simulink model "w2_warplab_buffers"  (Simulink 7.7)
settings: Solver=VariableStepDiscrete  SolverMode=SingleTasking  StartTime=0.0  StopTime=200000  RelTol=1e-3
InitFcn:
  | w2_warplab_buffers_init
StartFcn:
  | w2_warplab_buffers_init
values from neighbouring files (symbols this model uses):
  NumSamps_Rx_IQ = 2^14    (= 16384)    [w2_warplab_buffers_init.m]
  NumSamps_Rx_RSSI = 2^12    (= 4096)    [w2_warplab_buffers_init.m]
  NumSamps_Tx_IQ = 2^14    (= 16384)    [w2_warplab_buffers_init.m]
undefined symbols (not defined in the file or in its folder): gcbh, xlBlockLoadCallback, xlGetNormalizedPeriod
libraries: xbsIndex_r4 x752
(part 1 of 7)
settings Model: Creator=mduarte  LastModifiedBy=mango
settings OptimizationCC: InlineParams=on  InitFltsAndDblsToZero=on
settings DebuggingCC: SaveWithParameterizedLinksMsg=none  StrictBusMsg=Warning
settings GRTTargetCC: TargetFcnLib=ansi_tfl_tmw.mat

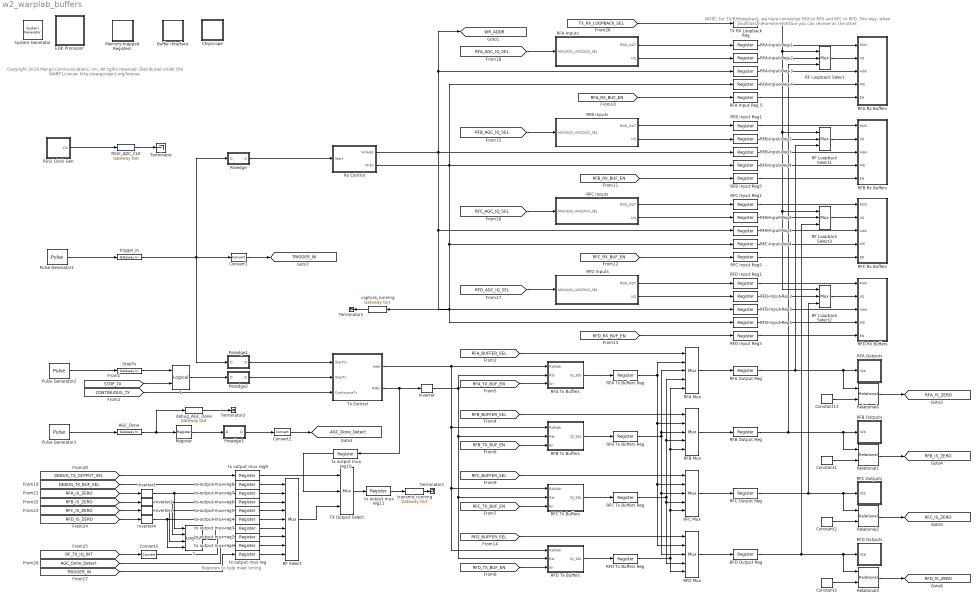
== system w2_warplab_buffers ==
  note: Copyright 2014 Mango Communications, Inc. All rights reserved.
      |
      | Distributed under the WARP License:
      | http://warpproject.org/license
  note: NOTE: For TX/RX Loopback, we have connected RFA to RFB and RFC to RFD.
      | This way, when you transmit on one interface you can receive on the other.
  note: Registers to help
      | meet timing
  " 1" : xbsIndex_r4/Logical  logical_function=OR  inputs=2  en=off  latency=0  precision=Full  arith_type=Unsigned  n_bits=16  bin_pt=0  align_bp=on  dbl_ovrd=off  block_type=logical
      settings: block_version=9.1.01
  " 2" : xbsIndex_r4/Logical  logical_function=OR  inputs=4  en=off  latency=0  precision=Full  arith_type=Unsigned  n_bits=16  bin_pt=0  align_bp=on  dbl_ovrd=off  block_type=logical
      settings: block_version=9.1.01
  " System Generator" : xbsIndex_r4/ System Generator  Tag=genX  SystemSampleTime=-1  xilinxfamily=virtex4  part=xc4vfx100  speed=-11  package=ff1517  synthesis_tool=XST  clock_wrapper=Clock Enables  directory=./warplab_buffers  proj_type=Project Navigator  Synth_file=XST Defaults  Impl_file=ISE Defaults  testbench=off  simulink_period=1  sysclk_period=10  dcm_input_clock_period=10  incr_netlist=off  trim_vbits=Everywhere in SubSystem  dbl_ovrd=According to Block Masks  core_generation=According to Block Masks  run_coregen=off  deprecated_control=off  eval_field=0  block_type=sysgen
  AGC_Done : xbsIndex_r4/Gateway In  gui_display_data_type=Fixed-point  arith_type=Unsigned  n_bits=1  bin_pt=0  preci_type=Single  exp_width=8  frac_width=24  quantization="Round  (unbiased: +/- Inf)"  overflow=Saturate  period=1  dbl_ovrd=off  timing_constraint=None  locs_specified=off  LOCs={}  UseAsADC=off  ADCChannel='1'  inherit_from_input=off  hdl_port=on  block_type=gatewayin
      settings: infoedit="Gateway in block.  Converts inputs of type Simulink integer, double and fixed point to  Xilinx fixed point type.<P><P>Hardware notes:  In hardware these blocks become top level input ports."  block_version=VER_STRING_GOES_HERE
  Buffer Interface : Subsystem
  Chipscope : Subsystem
  Constant{1..3,13} (4 alike) : xbsIndex_r4/Constant  const=0  gui_display_data_type=Fixed-point  arith_type=Unsigned  n_bits=32  bin_pt=0  preci_type=Single  exp_width=8  frac_width=24  explicit_period=off  period=1  equ=P=C  opselect=C  inp2=PCIN>>17  opr=+  inp1=P  carry=CIN  dbl_ovrd=off  block_type=constant
      settings: block_version=10.1.2
  Convert1 : xbsIndex_r4/Convert  gui_display_data_type=Boolean  arith_type=Boolean  n_bits=16  bin_pt=14  float_type=Single  exp_bits=8  fraction_bits=24  quantization=Truncate  overflow=Wrap  en=off  latency=0  dbl_ovrd=off  pipeline=off  block_type=convert
      settings: block_version=8.2
  Convert2 : xbsIndex_r4/Convert  gui_display_data_type=Fixed-point  arith_type=Boolean  n_bits=16  bin_pt=14  float_type=Single  exp_bits=8  fraction_bits=24  quantization=Truncate  overflow=Wrap  en=off  latency=0  dbl_ovrd=off  pipeline=off  block_type=convert
      settings: block_version=8.2
  Convert3 : xbsIndex_r4/Convert  gui_display_data_type=Fixed-point  arith_type=Boolean  n_bits=16  bin_pt=14  float_type=Single  exp_bits=8  fraction_bits=24  quantization=Truncate  overflow=Wrap  en=off  latency=0  dbl_ovrd=off  pipeline=off  block_type=convert
      settings: block_version=8.2
  EDK Processor : Subsystem  LoadFcn=xlBlockLoadCallback(gcbh);  mask(Xilinx EDK Processor Block){mode=EDK pcore generation, xmp=, MemVisToProc=<qt bgcolor="#FFFFFF"><div><img src="C:/Xilinx/14.4/ISE_DS/ISE/sysgen/data/images/registerplus.gif"> &lt;&lt;TX_DELAY&gt;&gt;<br></div><div><img src="C:/Xilinx/14.4/ISE_DS/ISE/sysgen/data/images/registerplus.gif"> &lt;&lt;RF_RX_IQ_BUF_RD_BYTE_OFFSET&gt;&gt;<br></div><div><img src="C:/Xilinx/14.4/ISE_DS/ISE/sysgen/data/images/registerplus.gif"> &lt;&lt;LOAD_TIMER_64_LSB&gt;&gt;<br></div><div><img src="C:/Xilinx/14.4/ISE_DS/ISE/sysgen/data/images/registerplus.gif"> &lt;&lt;RF_RX_IQ_THRESHOLD&gt;&gt;<br></div><div><img src="C:/Xilinx/14.4/ISE_DS/ISE/sysgen/data/images/registerplus.gif"> &lt;&lt;RX_LENGTH&gt;&gt;<br></div><div><img src="C:/Xilinx/14.4/ISE_DS/ISE/sysgen/data/images/registerplus.gif"> &lt;&lt;TX_LENGTH&gt;&gt;<br></div><div><img src="C:/Xilinx/14.4/ISE_DS/ISE/sysgen/data/images/registerplus.gif"> &lt;&lt;RF_RX_IQ_BUF_WR_BYTE_OFFSET&gt;&gt;<br></div><div><img src="C:/Xilinx/14.4/ISE_DS/ISE/sysgen/data/images/registerplus.gif"> &lt;&lt;RF_BUFFER_SEL&gt;&gt;<br></div><div><img src="C:/Xilinx/14.4/ISE_DS/ISE/sysgen/data/images/registerplus.gif"> &lt;&lt;RX_BUF_EN&gt;&gt;<br></div><div><img src="C:/Xilinx/14.4/ISE_DS/ISE/sysgen/data/images/registerplus.gif"> &lt;&lt;RF_TX_IQ_THRESHOLD&gt;&gt;<br></div><div><img src="C:/Xilinx/14.4/ISE_DS/ISE/sysgen/data/images/registerplus.gif"> &lt;&lt;CONFIG&gt;&gt;<br></div><div><img src="C:/Xilinx/14.4/ISE_DS/ISE/sysgen/data/images/registerplus.gif"> &lt;&lt;RF_ERROR_CLR&gt;&gt;<br></div><div><img src="C:/Xilinx/14.4/ISE_DS/ISE/sysgen/data/images/registerplus.gif"> &lt;&lt;RF_TX_IQ_BUF_WR_BYTE_OFFSET&gt;&gt;<br></div><div><img src="C:/Xilinx/14.4/ISE_DS/ISE/sysgen/data/images/registerplus.gif"> &lt;&lt;LOAD_TIMER_64_MSB&gt;&gt;<br></div><div><img src="C:/Xilinx/14.4/ISE_DS/ISE/sysgen/data/images/registerplus.gif"> &lt;&lt;TX_BUF_EN&gt;&gt;<br></div><div><img src="C:/Xilinx/14.4/ISE_DS/ISE/sysgen/data/images/registerplus.gif"> &lt;&lt;RF_TX_IQ_BUF_OCCUPANCY&gt;&gt;<br></div><div><img src="C:/Xilinx/14.4/ISE_DS/ISE/sysgen/data/images/registerplus.gif"> &lt;&lt;RF_TX_IQ_BUF_RD_BYTE_OFFSET&gt;&gt;<br></div><div><img src="C:/Xilinx/14.4/ISE_DS/ISE/sysgen/data/images/registerplus.gif"> &lt;&lt;AGC_GAINS&gt;&gt;<br></div><div><img src="C:/Xilinx/14.4/ISE_DS/ISE/sysgen/data/images/registerplus.gif"> &lt;&lt;RF_RX_IQ_BUF_OCCUPANCY&gt;&gt;<br></div><div><img src="C:/Xilinx/14.4/ISE_DS/ISE/sysgen/data/images/registerplus.gif"> &lt;&lt;RF_RX_IQ_BUF_WR_BYTE_OFFSET_UPDATE&gt;&gt;<br></div><div><img src="C:/Xilinx/14.4/ISE_DS/ISE/sysgen/data/images/registerplus.gif"> &lt;&lt;INT_STATUS&gt;&gt;<br></div><div><img src="C:/Xilinx/14.4/ISE_DS/ISE/sysgen/data/images/registerplus.gif"> &lt;&lt;BUFF_SIZES&gt;&gt;<br></div><div><img src="C:/Xilinx/14.4/ISE_DS/ISE/sysgen/data/images/registerplus.gif"> &lt;&lt;DESIGN_VER&gt;&gt;<br></div><div><img src="C:/Xilinx/14.4/ISE_DS/ISE/sysgen/data/images/registerplus.gif"> &lt;&lt;RF_TX_IQ_STATUS&gt;&gt;<br></div><div><img src="C:/Xilinx/14.4/ISE_DS/ISE/sysgen/data/images/registerplus.gif"> &lt;&lt;STATUS&gt;&gt;<br></div><div><img src="C:/Xilinx/14.4/ISE_DS/ISE/sysgen/data/images/registerplus.gif"> &lt;&lt;RFCD_AGC_DONE_RSSI&gt;&gt;<br></div><div><img src="C:/Xilinx/14.4/ISE_DS/ISE/sysgen/data/images/registerplus.gif"> &lt;&lt;RFAB_AGC_DONE_RSSI&gt;&gt;<br></div><div><img src="C:/Xilinx/14.4/ISE_DS/ISE/sysgen/data/images/registerplus.gif"> &lt;&lt;TIMER_64_MSB&gt;&gt;<br></div><div><img src="C:/Xilinx/14.4/ISE_DS/ISE/sysgen/data/images/registerplus.gif"> &lt;&lt;TIMER_64_LSB&gt;&gt;<br></div><div><img src="C:/Xilinx/14.4/ISE_DS/ISE/sysgen/data/images/registerplus.gif"> &lt;&lt;AGC_DONE_ADDR&gt;&gt;<br></div><div><img src="C:/Xilinx/14.4/ISE_DS/ISE/sysgen/data/images/memoryplus.gif"> &lt;&lt;RFD_IQ_Tx_Buffer&gt;&gt;<br></div><div><img src="C:/Xilinx/14.4/ISE_DS/ISE/sysgen/data/images/memoryplus.gif"> &lt;&lt;RFD_RSSI_Buffer&gt;&gt;<br></div><div><img src="C:/Xilinx/14.4/ISE_DS/ISE/sysgen/data/images/memoryplus.gif"> &lt;&lt;RFD_IQ_Rx_Buffer&gt;&gt;<br></div><div><img src="C:/Xilinx/14.4/ISE_DS/ISE/sysgen/data/images/memoryplus.gif"> &lt;&lt;RFC_IQ_Tx_Buffer&gt;&gt;<br></div><div><img src="C:/Xilinx/14.4/ISE_DS/ISE/sysgen/data/images/memoryplus.gif"> &lt;&lt;RFC_RSSI_Buffer&gt;&gt;<br></div><div><img src="C:/Xilinx/14.4/ISE_DS/ISE/sysgen/data/images/memoryplus.gif"> &lt;&lt;RFC_IQ_Rx_Buffer&gt;&gt;<br></div><div><img src="C:/Xilinx/14.4/ISE_DS/ISE/sysgen/data/images/memoryplus.gif"> &lt;&lt;RFB_IQ_Tx_Buffer&gt;&gt;<br></div><div><img src="C:/Xilinx/14.4/ISE_DS/ISE/sysgen/data/images/memoryplus.gif"> &lt;&lt;RFB_RSSI_Buffer&gt;&gt;<br></div><div><img src="C:/Xilinx/14.4/ISE_DS/ISE/sysgen/data/images/memoryplus.gif"> &lt;&lt;RFB_IQ_Rx_Buffer&gt;&gt;<br></div><div><img src="C:/Xilinx/14.4/ISE_DS/ISE/sysgen/data/images/memoryplus.gif"> &lt;&lt;RFA_IQ_Tx_Buffer&gt;&gt;<br></div><div><img src="C:/Xilinx/14.4/ISE_DS/ISE/sysgen/data/images/memoryplus.gif"> &lt;&lt;RFA_RSSI_Buffer&gt;&gt;<br></div><div><img src="C:/Xilinx/14.4/ISE_DS/ISE/sysgen/data/images/memoryplus.gif"> &lt;&lt;RFA_IQ_Rx_Buffer&gt;&gt;<br></div></qt>, AvailableMemories=<empty>, portInterfaceTable={'exposed'=>[],'portdir'=>[],'portname'=>[],'shortname'=>[]}, bus_type_sgadvanced=, bus_type=PLB, baseaddr=0x80000000, baseaddr_lock_sgadvanced=, baseaddr_lock=off, dual_clock_sgadvanced=, dual_clock=on, reg_readback_sgadvanced=, reg_readback=on, ucf_file=, inheritDeviceType_sgadvanced=, inheritDeviceType=off, elf_file=, codebug_sgadvanced=, codebug=on, clock_name=plb, internalPortList={}, resetPolarity=0, memxtable={'mladdr'=>[0.00000000000000000,1.00000000000000000,2.00000000000000000,3.00000000000000000,4.00000000000000000,5.00000000000000000,6.00000000000000000,7.00000000000000000,8.00000000000000000,9.00000000000000000,10.00000000000000000,11.00000000000000000,12.00000000000000000,13.00000000000000000,14.00000000000000000,0.00000000000000000,1.00000000000000000,2.00000000000000000,3.00000000000000000,4.00000000000000000,5.00000000000000000,6.00000000000000000,7.00000000000000000,8.00000000000000000,9.00000000000000000,10.00000000000000000,11.00000000000000000,12.00000000000000000,13.00000000000000000,14.00000000000000000,-1.00000000000000000,-1.00000000000000000,-1.00000000000000000,-1.00000000000000000,-1.00000000000000000,-1.00000000000000000,-1.00000000000000000,-1.00000000000000000,-1.00000000000000000,-1.00000000000000000,-1.00000000000000000,-1.00000000000000000],'mlist'=>['w2_warplab_buffers/Memory-mapped Registers/TxDelay','w2_warplab_buffers/Memory-mapped Registers/From Register9','w2_warplab_buffers/Memory-mapped Registers/From Register8','w2_warplab_buffers/Memory-mapped Registers/From Register7','w2_warplab_buffers/Memory-mapped Registers/From Register6','w2_warplab_buffers/Memory-mapped Registers/From Register5','w2_warplab_buffers/Memory-mapped Registers/From Register4','w2_warplab_buffers/Memory-mapped Registers/From Register2','w2_warplab_buffers/Memory-mapped Registers/From Register16','w2_warplab_buffers/Memory-mapped Registers/From Register14','w2_warplab_buffers/Memory-mapped Registers/From Register13','w2_warplab_buffers/Memory-mapped Registers/From Register12','w2_warplab_buffers/Memory-mapped Registers/From Register11','w2_warplab_buffers/Memory-mapped Registers/From Register10','w2_warplab_buffers/Memory-mapped Registers/From Register1','w2_warplab_buffers/Memory-mapped Registers/To Register9','w2_warplab_buffers/Memory-mapped Registers/To Register8','w2_warplab_buffers/Memory-mapped Registers/To Register7','w2_warplab_buffers/Memory-mapped Registers/To Register6','w2_warplab_buffers/Memory-mapped Registers/To Register5','w2_warplab_buffers/Memory-mapped Registers/To Register4','w2_warplab_buffers/Memory-mapped Registers/To Register3','w2_warplab_buffers/Memory-mapped Registers/To Register2','w2_warplab_buffers/Memory-mapped Registers/To Register10','w2_warplab_buffers/Memory-mapped Registers/To Register1','w2_warplab_buffers/Memory-mapped Registers/Radio3AGCDoneRSSI','w2_warplab_buffers/Memory-mapped Registers/Radio1AGCDoneRSSI','w2_warplab_buffers/Memory-mapped Registers/AGCDoneAddr2','w2_warplab_buffers/Memory-mapped Registers/AGCDoneAddr1','w2_warplab_buffers/Memory-mapped Registers/AGCDoneAddr','w2_warplab_buffers/Buffer Interface/RFD Buffers/Shared Memory2','w2_warplab_buffers/Buffer Interface/RFD Buffers/Shared Memory1','w2_warplab_buffers/Buffer Interface/RFD Buffers/Shared Memory','w2_warplab_buffers/Buffer Interface/RFC Buffers/Shared Memory2','w2_warplab_buffers/Buffer Interface/RFC Buffers/Shared Memory1','w2_warplab_buffers/Buffer Interface/RFC Buffers/Shared Memory','w2_warplab_buffers/Buffer Interface/RFB Buffers/Shared Memory2','w2_warplab_buffers/Buffer Interface/RFB Buffers/Shared Memory1','w2_warplab_buffers/Buffer Interface/RFB Buffers/Shared Memory','w2_warplab_buffers/Buffer Interface/RFA Buffers/Shared Memory2','w2_warplab_buffers/Buffer Interface/RFA Buffers/Shared Memory1','w2_warplab_buffers/Buffer Interface/RFA Buffers/Shared Memory'],'mlname'=>['\\'TX_DELAY\\'','\\'RF_RX_IQ_BUF_RD_BYTE_OFFSET\\'','\\'LOAD_TIMER_64_LSB\\'','\\'RF_RX_IQ_THRESHOLD\\'','\\'RX_LENGTH\\'','\\'TX_LENGTH\\'','\\'RF_RX_IQ_BUF_WR_BYTE_OFFSET\\'','\\'RF_BUFFER_SEL\\'','\\'RX_BUF_EN\\'','\\'RF_TX_IQ_THRESHOLD\\'','\\'CONFIG\\'','\\'RF_ERROR_CLR\\'','\\'RF_TX_IQ_BUF_WR_BYTE_OFFSET\\'','\\'LOAD_TIMER_64_MSB\\'','\\'TX_BUF_EN\\'','\\'RF_TX_IQ_BUF_OCCUPANCY\\'','\\'RF_TX_IQ_BUF_RD_BYTE_OFFSET\\'','\\'AGC_GAINS\\'','\\'RF_RX_IQ_BUF_OCCUPANCY\\'','\\'RF_RX_IQ_BUF_WR_BYTE_OFFSET_UPDATE\\'','\\'INT_STATUS\\'','\\'BUFF_SIZES\\'','\\'DESIGN_VER\\'','\\'RF_TX_IQ_STATUS\\'','\\'STATUS\\'','\\'RFCD_AGC_DONE_RSSI\\'','\\'RFAB_AGC_DONE_RSSI\\'','\\'TIMER_64_MSB\\'','\\'TIMER_64_LSB\\'','\\'AGC_DONE_ADDR\\'','\\'RFD_IQ_Tx_Buffer\\'','\\'RFD_RSSI_Buffer\\'','\\'RFD_IQ_Rx_Buffer\\'','\\'RFC_IQ_Tx_Buffer\\'','\\'RFC_RSSI_Buffer\\'','\\'RFC_IQ_Rx_Buffer\\'','\\'RFB_IQ_Tx_Buffer\\'','\\'RFB_RSSI_Buffer\\'','\\'RFB_IQ_Rx_Buffer\\'','\\'RFA_IQ_Tx_Buffer\\'','\\'RFA_RSSI_Buffer\\'','\\'RFA_IQ_Rx_Buffer\\''],'mlstate'=>[0.00000000000000000,0.00000000000000000,0.00000000000000000,0.00000000000000000,0.00000000000000000,0.00000000000000000,0.00000000000000000,0.00000000000000000,0.00000000000000000,0.00000000000000000,0.00000000000000000,0.00000000000000000,0.00000000000000000,0.00000000000000000,0.00000000000000000,0.00000000000000000,0.00000000000000000,0.00000000000000000,0.00000000000000000,0.00000000000000000,0.00000000000000000,0.00000000000000000,0.00000000000000000,0.00000000000000000,0.00000000000000000,0.00000000000000000,0.00000000000000000,0.00000000000000000,0.00000000000000000,0.00000000000000000,0.00000000000000000,0.00000000000000000,0.00000000000000000,0.00000000000000000,0.00000000000000000,0.00000000000000000,0.00000000000000000,0.00000000000000000,0.00000000000000000,0.00000000000000000,0.00000000000000000,0.00000000000000000]}, procinfo={}, memmapdirty=off, blockname=, xpsintstyle=default, has_advanced_control=0, sggui_pos=-1,-1,-1,-1, block_type=edkprocessor, block_version=2.7, sg_icon_stat=62,64,-1,-1,white,blue,0,07734,right,,[ ],[ ], sg_mask_display=|, sg_list_contents={'table'=>{'AvailableMemories'=>'popup(<empty>)'}}, sg_blockgui_xml=}
      mask sg_mask_display=|
      | fprintf('','COMMENT: begin icon graphics');
      | patch([0 62 62 0 0 ],[0 0 64 64 0 ],[0.77 0.82 0.91 ]);
      | plot([0 62 62 0 0 ],[0 0 64 64 0 ]);
      | patch([13.2 24.76 32.76 40.76 48.76 32.76 21.2 13.2 ],[40.88 40.88 48.88 40.88 48.88 48.88 48.88 40.88 ],[1 1 1 ]);
      | patch([21.2 32.76 24.76 13.2 21.2 ],[32.88 32.88 40.88 40.88 32.88 ],[0.931 0.946 0.973 ]);
      | patch([13.2 24.76 32.76 21.2 13.2 ],[24.88 24.88 32.88 32.88 24.88 ],[1 1 1 ]);
      | patch([21.2 48.76 40.76 32.76 24.76 13.2 21.2 ],[16.88 16.88 24.88 16.88 24.88 24.88 16.88 ],[0.931 0.946 0.973 ]);
      | fprintf('','COMMENT: end icon graphics');
      | fprintf('','COMMENT: begin icon text');
      | fprintf('','COMMENT: end icon text');
      mask prompts: mode "Configure Processor for"; xmp "XPS Project"; MemVisToProc ""; AvailableMemories "Available Memories"; portInterfaceTable ""; bus_type_sgadvanced ""; bus_type "Bus Type"; baseaddr "Base Address"; baseaddr_lock_sgadvanced ""; baseaddr_lock "Lock"; dual_clock_sgadvanced ""; dual_clock "Dual Clocks"; reg_readback_sgadvanced ""; reg_readback "Register Read-Back"; ucf_file "Constraint File"; inheritDeviceType_sgadvanced ""; inheritDeviceType "Inherit Device Type"; elf_file "Initial Program"; codebug_sgadvanced ""; codebug "Enable Co-Debug with Xilinx SDK (Beta)"; clock_name ""; internalPortList ""; resetPolarity ""; memxtable ""; procinfo ""; memmapdirty ""; blockname ""; xpsintstyle ""; has_advanced_control ""; sggui_pos ""; block_type ""; block_version ""; sg_icon_stat ""; sg_mask_display ""; sg_list_contents ""; sg_blockgui_xml ""
      mask help: Xilinx EDK Processor
      mask init:
      | try
      |   tmp_gcb = gcb;
      |   tmp_gcbh = gcbh;
      |   if (strcmp('SysGenIndex',get_param(bdroot(tmp_gcbh),'tag')) && ~isempty(regexp(bdroot(tmp_gcb), '^xbs', 'once')))
      |     return;
      |   end;
      |   xlMungeMaskParams;
      | 
      |   block_type='edkprocessor';
      | 
      |   serialized_declarations = '{''block_type''=>''String''}';
      |   xledkprocessor_init();
      |   ptable_ = xlblockprep(get_param(tmp_gcb, 'MaskWSVariables'));
      |   try
      |     xlBlockMoveCallback(tmp_gcbh);
      |   catch 
      |      clear global xl_updateicon_recursion_guard;
      |   end;
      | catch
      |   global dbgsysgen;
      |   if(~isempty(dbgsysgen) && dbgsysgen)
      |     e = regexprep(lasterr, '\n', '\nError: ');
      |     disp(['Error: While running MaskInit code on block ' tmp_gcb ': ' e]);
      |     error(e);
      |   end
      | end
      settings: CopyFcn=xlProcBlockCopyCallback(gcbh);xlBlockMoveCallback(gcbh);  DeleteFcn=xlDestroyGui(gcbh);  ModelCloseFcn=xlDestroyGui(gcbh);  PreSaveFcn=xlBlockPreSaveCallback(gcbh);  PostSaveFcn=xlBlockPostSaveCallback(gcbh);  DestroyFcn=xlDestroyGui(gcbh);  OpenFcn=bh=gcbh;xlProcBlockCallbacks('populatesharedmemorylistbox',bh);xlOpenGui(bh, 'edkprocessor_gui.xml', @xlProcBlockEnablement, @xlProcBlockAction);  CloseFcn=xlDestroyGui(gcbh);  MoveFcn=xlBlockMoveCallback(gcbh);
      mask Help: eval('');xlDoc('-book','sysgen','-topic','EDK_Processor');
      mask StyleString: popup(EDK pcore generation|HDL netlisting),edit,edit,edit,edit,edit,popup(AXI|PLB),edit,edit,checkbox,edit,checkbox,edit,checkbox,edit,edit,checkbox,edit,edit,checkbox,edit,edit,edit,edit,edit,edit,edit,edit,edit,edit,edit,edit,edit,edit,edit,edit
      mask Display:
      | fprintf('','COMMENT: begin icon graphics');
      | patch([0 62 62 0 0 ],[0 0 64 64 0 ],[0.77 0.82 0.91 ]);
      | plot([0 62 62 0 0 ],[0 0 64 64 0 ]);
      | patch([13.2 24.76 32.76 40.76 48.76 32.76 21.2 13.2 ],[40.88 40.88 48.88 40.88 48.88 48.88 48.88 40.88 ],[1 1 1 ]);
      | patch([21.2 32.76 24.76 13.2 21.2 ],[32.88 32.88 40.88 40.88 32.88 ],[0.931 0.946 0.973 ]);
      | patch([13.2 24.76 32.76 21.2 13.2 ],[24.88 24.88 32.88 32.88 24.88 ],[1 1 1 ]);
      | patch([21.2 48.76 40.76 32.76 24.76 13.2 21.2 ],[16.88 16.88 24.88 16.88 24.88 24.88 16.88 ],[0.931 0.946 0.973 ]);
      | fprintf('','COMMENT: end icon graphics');
      | fprintf('','COMMENT: begin icon text');
      | disp('');
      | 
      | fprintf('','COMMENT: end icon text');
  Inverter{,1..4} (5 alike) : xbsIndex_r4/Inverter  en=off  latency=0  dbl_ovrd=off  block_type=inv
      settings: block_version=8.2
  Memory-mapped Registers : Subsystem
  Posedge : Subsystem
  Posedge1 : Subsystem
  Posedge2 : Subsystem
  Posedge3 : Subsystem
  Pulse Generator1 : DiscretePulseGenerator  Period=2^20  PulseWidth=50  PhaseDelay=100
  Pulse Generator2 : DiscretePulseGenerator  Period=10 * 2^14  PulseWidth=50  PhaseDelay=2.5 * 2^14
  Pulse Generator3 : DiscretePulseGenerator  Period=20000  PulseWidth=50  PhaseDelay=374
  RF Loopback Select{,1..3} (4 alike) : xbsIndex_r4/Mux  inputs=2  en=off  latency=0  precision=Full  arith_type=Unsigned  n_bits=16  bin_pt=14  quantization=Truncate  overflow=Wrap  dbl_ovrd=off  block_type=mux
  RF Select : xbsIndex_r4/Mux  inputs=8  en=off  latency=0  precision=Full  arith_type=Unsigned  n_bits=16  bin_pt=14  quantization=Truncate  overflow=Wrap  dbl_ovrd=off  block_type=mux
  RFA Rx Buffers : Subsystem
  RFA Input Reg {1..5} (5 alike) : xbsIndex_r4/Register  init=0  rst=off  en=off  dbl_ovrd=off  block_type=register
  RFA Inputs : Subsystem
  RFA Mux : xbsIndex_r4/Mux  inputs=4  en=off  latency=0  precision=Full  arith_type=Unsigned  n_bits=16  bin_pt=14  quantization=Truncate  overflow=Wrap  dbl_ovrd=off  block_type=mux
  "RFA Output Reg " : xbsIndex_r4/Register  init=0  rst=off  en=off  dbl_ovrd=off  block_type=register
  RFA Outputs : Subsystem
  RFA Tx Buffers : Subsystem
  RFA Tx Buffers Reg : xbsIndex_r4/Register  init=0  rst=off  en=off  dbl_ovrd=off  block_type=register
  RFB Rx Buffers : Subsystem
  RFB Input Reg{1..5} (5 alike) : xbsIndex_r4/Register  init=0  rst=off  en=off  dbl_ovrd=off  block_type=register
  RFB Inputs : Subsystem
  RFB Mux : xbsIndex_r4/Mux  inputs=4  en=off  latency=0  precision=Full  arith_type=Unsigned  n_bits=16  bin_pt=14  quantization=Truncate  overflow=Wrap  dbl_ovrd=off  block_type=mux
  RFB Output Reg : xbsIndex_r4/Register  init=0  rst=off  en=off  dbl_ovrd=off  block_type=register
  RFB Outputs : Subsystem
  RFB Tx Buffers : Subsystem
  RFB Tx Buffers Reg : xbsIndex_r4/Register  init=0  rst=off  en=off  dbl_ovrd=off  block_type=register
  RFC Rx Buffers : Subsystem
  RFC Input Reg{1..5} (5 alike) : xbsIndex_r4/Register  init=0  rst=off  en=off  dbl_ovrd=off  block_type=register
  RFC Inputs : Subsystem
  RFC Mux : xbsIndex_r4/Mux  inputs=4  en=off  latency=0  precision=Full  arith_type=Unsigned  n_bits=16  bin_pt=14  quantization=Truncate  overflow=Wrap  dbl_ovrd=off  block_type=mux
  RFC Output Reg : xbsIndex_r4/Register  init=0  rst=off  en=off  dbl_ovrd=off  block_type=register
  RFC Outputs : Subsystem
  RFC Tx Buffers : Subsystem
  RFC Tx Buffers Reg : xbsIndex_r4/Register  init=0  rst=off  en=off  dbl_ovrd=off  block_type=register
  RFD Rx Buffers : Subsystem
  RFD Input Reg{1..5} (5 alike) : xbsIndex_r4/Register  init=0  rst=off  en=off  dbl_ovrd=off  block_type=register
  RFD Inputs : Subsystem
  RFD Mux : xbsIndex_r4/Mux  inputs=4  en=off  latency=0  precision=Full  arith_type=Unsigned  n_bits=16  bin_pt=14  quantization=Truncate  overflow=Wrap  dbl_ovrd=off  block_type=mux
  RFD Output Reg : xbsIndex_r4/Register  init=0  rst=off  en=off  dbl_ovrd=off  block_type=register
  RFD Outputs : Subsystem
  RFD Tx Buffers : Subsystem
  RFD Tx Buffers Reg : xbsIndex_r4/Register  init=0  rst=off  en=off  dbl_ovrd=off  block_type=register
  RSSI Clock Gen : Subsystem
  RSSI_ADC_CLK : xbsIndex_r4/Gateway Out  inherit_from_input=off  hdl_port=on  timing_constraint=None  locs_specified=off  LOCs={}  UseAsDAC=off  DACChannel='1'  block_type=gatewayout
      settings: infoedit="Gateway out block.  Converts Xilinx fixed point inputs into ouputs of type Simulink integer, double, or fixed point.<P><P>Hardware notes:  In hardware these blocks become top level output ports or are discarded, depending on how they are configured."  block_version=8.2
  Register : xbsIndex_r4/Register  init=0  rst=off  en=off  dbl_ovrd=off  block_type=register
      settings: block_version=8.2
  Relational{1..3,6} (4 alike) : xbsIndex_r4/Relational  mode=a=b  en=off  latency=0  dbl_ovrd=off  block_type=relational
      settings: block_version=8.2
  Rx Control : Subsystem
  StopTx : xbsIndex_r4/Gateway In  gui_display_data_type=Fixed-point  arith_type=Unsigned  n_bits=1  bin_pt=0  preci_type=Single  exp_width=8  frac_width=24  quantization="Round  (unbiased: +/- Inf)"  overflow=Saturate  period=1  dbl_ovrd=off  timing_constraint=None  locs_specified=off  LOCs={}  UseAsADC=off  ADCChannel='1'  inherit_from_input=off  hdl_port=on  block_type=gatewayin
      settings: block_version=VER_STRING_GOES_HERE
  TX Output Select : xbsIndex_r4/Mux  inputs=2  en=off  latency=0  precision=Full  arith_type=Unsigned  n_bits=16  bin_pt=14  quantization=Truncate  overflow=Wrap  dbl_ovrd=off  block_type=mux
  TX RX Loopback Reg : xbsIndex_r4/Register  init=0  rst=off  en=off  dbl_ovrd=off  block_type=register
  Terminator{,1..3} (4 alike) : Terminator
  Tx Control : Subsystem
  capture_running : xbsIndex_r4/Gateway Out  inherit_from_input=off  hdl_port=on  timing_constraint=None  locs_specified=off  LOCs={}  UseAsDAC=off  DACChannel='1'  block_type=gatewayout
      settings: infoedit="Gateway out block.  Converts Xilinx fixed point inputs into ouputs of type Simulink integer, double, or fixed point.<P><P>Hardware notes:  In hardware these blocks become top level output ports or are discarded, depending on how they are configured."  block_version=8.2
  debug_AGC_Done : xbsIndex_r4/Gateway Out  inherit_from_input=off  hdl_port=on  timing_constraint=None  locs_specified=off  LOCs={}  UseAsDAC=off  DACChannel='1'  block_type=gatewayout
      settings: block_version=8.2
  transmit_running : xbsIndex_r4/Gateway Out  inherit_from_input=off  hdl_port=on  timing_constraint=None  locs_specified=off  LOCs={}  UseAsDAC=off  DACChannel='1'  block_type=gatewayout
      settings: infoedit="Gateway out block.  Converts Xilinx fixed point inputs into ouputs of type Simulink integer, double, or fixed point.<P><P>Hardware notes:  In hardware these blocks become top level output ports or are discarded, depending on how they are configured."  block_version=8.2
  trigger_in : xbsIndex_r4/Gateway In  gui_display_data_type=Fixed-point  arith_type=Unsigned  n_bits=1  bin_pt=0  preci_type=Single  exp_width=8  frac_width=24  quantization="Round  (unbiased: +/- Inf)"  overflow=Saturate  period=1  dbl_ovrd=off  timing_constraint=None  locs_specified=off  LOCs={}  UseAsADC=off  ADCChannel='1'  inherit_from_input=off  hdl_port=on  block_type=gatewayin
      settings: infoedit="Gateway in block.  Converts inputs of type Simulink integer, double and fixed point to  Xilinx fixed point type.<P><P>Hardware notes:  In hardware these blocks become top level input ports."  block_version=VER_STRING_GOES_HERE
  tx output mux reg{,1..11} (12 alike) : xbsIndex_r4/Register  init=0  rst=off  en=off  dbl_ovrd=off  block_type=register
  tag scope: AGC_Done_Detect=global, RFA_IS_ZERO=global, RFB_IS_ZERO=global, RFC_IS_ZERO=global, RFD_IS_ZERO=global, TRIGGER_IN=global, WR_ADDR=global
  wires:
  [RFC_RX_BUF_EN] -> RFC Input Reg5/1
  [RFB_RX_BUF_EN] -> RFB Input Reg5/1
  Posedge/1(Q) -> Rx Control/1(Start)
  [RFA_RX_BUF_EN] -> RFA Input Reg 5/1
  [RFD_RX_BUF_EN] -> RFD Input Reg5/1
  Rx Control/1(WrAddr) -> RFC Input Reg3/1, RFD Input Reg3/1, [WR_ADDR], RFA Input Reg 3/1, RFB Input Reg3/1
  Rx Control/2(WrEn) -> capture_running/1, RFD Input Reg4/1, RFC Input Reg4/1, RFB Input Reg4/1, RFA Input Reg 4/1
  Posedge1/1(Q) -> Tx Control/1(StartTx)
  [CONTINUOUS_TX] -> Tx Control/3(ContinuousTx)
  Posedge2/1(Q) -> Tx Control/2(StopTx)
  " 1"/1 -> Posedge2/1(D)
  StopTx/1 -> " 1"/1
  Pulse Generator2/1 -> StopTx/1
  [RFB_TX_BUF_EN] -> RFB Tx Buffers/3(En)
  Tx Control/2(RdEn) -> Inverter/1, tx output mux reg10/1
  [RFC_TX_BUF_EN] -> RFC Tx Buffers/3(En)
  [RFA_TX_BUF_EN] -> RFA Tx Buffers/3(En)
  [RFD_TX_BUF_EN] -> RFD Tx Buffers/3(En)
  Tx Control/1(Addr) -> RFC Tx Buffers/1(RdAddr), RFD Tx Buffers/1(RdAddr), RFB Tx Buffers/1(RdAddr), RFA Tx Buffers/1(RdAddr)
  Inverter/1 -> RFC Tx Buffers/2(Rst), RFD Tx Buffers/2(Rst), RFB Tx Buffers/2(Rst), RFA Tx Buffers/2(Rst)
  [STOP_TX] -> " 1"/2
  AGC_Done/1 -> debug_AGC_Done/1, Register/1
  Pulse Generator3/1 -> AGC_Done/1
  Register/1 -> Posedge3/1(D)
  Posedge3/1(Q) -> Convert2/1
  Convert2/1 -> [AGC_Done_Detect]
  capture_running/1 -> Terminator2/1
  transmit_running/1 -> Terminator1/1
  RFA Inputs/1(RSSI_OUT) -> RFA Input Reg 1/1
  RFB Inputs/1(RSSI_OUT) -> RFB Input Reg1/1
  RFC Inputs/1(RSSI_OUT) -> RFC Input Reg1/1
  RFD Inputs/1(RSSI_OUT) -> RFD Input Reg1/1
  trigger_in/1 -> Posedge1/1(D), Posedge/1(D), Convert1/1
  RSSI_ADC_CLK/1 -> Terminator/1
  RSSI Clock Gen/1(Clk) -> RSSI_ADC_CLK/1
  Pulse Generator1/1 -> trigger_in/1
  RFA Tx Buffers/1(IQ_32b) -> RFA Tx Buffers Reg/1
  RFB Tx Buffers/1(IQ_32b) -> RFB Tx Buffers Reg/1
  RFC Tx Buffers/1(IQ_32b) -> RFC Tx Buffers Reg/1
  RFD Tx Buffers/1(IQ_32b) -> RFD Tx Buffers Reg/1
  "RFA Output Reg "/1 -> RFA Outputs/1(32b), Relational6/1, RF Loopback Select1/3
  RFB Output Reg/1 -> RFB Outputs/1(32b), Relational1/1, RF Loopback Select/3
  RFC Output Reg/1 -> RFC Outputs/1(32b), Relational2/1, RF Loopback Select2/3
  RFD Output Reg/1 -> RFD Outputs/1(32b), Relational3/1, RF Loopback Select3/3
  RFD Mux/1 -> RFD Output Reg/1
  RFC Mux/1 -> RFC Output Reg/1
  RFB Mux/1 -> RFB Output Reg/1
  RFA Mux/1 -> "RFA Output Reg "/1
  [RFA_BUFFER_SEL] -> RFA Mux/1
  [RFB_BUFFER_SEL] -> RFB Mux/1
  [RFC_BUFFER_SEL] -> RFC Mux/1
  [RFD_BUFFER_SEL] -> RFD Mux/1
  debug_AGC_Done/1 -> Terminator3/1
  [RFA_AGC_IQ_SEL] -> RFA Inputs/1(MGCAGC_AGCDCO_SEL)
  [RFB_AGC_IQ_SEL] -> RFB Inputs/1(MGCAGC_AGCDCO_SEL)
  [RFC_AGC_IQ_SEL] -> RFC Inputs/1(MGCAGC_AGCDCO_SEL)
  [RFD_AGC_IQ_SEL] -> RFD Inputs/1(MGCAGC_AGCDCO_SEL)
  Constant13/1 -> Relational6/2
  Relational6/1 -> [RFA_IS_ZERO]
  [DEBUG_TX_OUTPUT_SEL] -> tx output mux reg9/1
  RF Select/1 -> TX Output Select/3
  Constant1/1 -> Relational1/2
  Relational1/1 -> [RFB_IS_ZERO]
  Constant2/1 -> Relational2/2
  Relational2/1 -> [RFC_IS_ZERO]
  Constant3/1 -> Relational3/2
  Relational3/1 -> [RFD_IS_ZERO]
  [DEBUG_TX_BUF_SEL] -> tx output mux reg8/1
  [RFA_IS_ZERO] -> Inverter1/1
  [RFB_IS_ZERO] -> Inverter2/1
  [RFC_IS_ZERO] -> Inverter3/1
  [RFD_IS_ZERO] -> Inverter4/1
  Inverter1/1 -> " 2"/1, tx output mux reg7/1
  Inverter2/1 -> " 2"/2, tx output mux reg6/1
  Inverter3/1 -> " 2"/3, tx output mux reg5/1
  Inverter4/1 -> " 2"/4, tx output mux reg4/1
  RFA Tx Buffers Reg/1 -> RFA Mux/2, RFB Mux/2, RFC Mux/2, RFD Mux/2
  RFB Tx Buffers Reg/1 -> RFA Mux/3, RFC Mux/3, RFD Mux/3, RFB Mux/3
  RFC Tx Buffers Reg/1 -> RFA Mux/4, RFB Mux/4, RFC Mux/4, RFD Mux/4
  RFD Tx Buffers Reg/1 -> RFD Mux/5, RFC Mux/5, RFA Mux/5, RFB Mux/5
  " 2"/1 -> tx output mux reg3/1
  [RF_TX_IQ_INT] -> Convert3/1
  [AGC_Done_Detect] -> tx output mux reg1/1
  [TRIGGER_IN] -> tx output mux reg/1
  Convert1/1 -> [TRIGGER_IN]
  [TX_RX_LOOPBACK_SEL] -> TX RX Loopback Reg/1
  RFA Inputs/2(I/Q) -> RFA Input Reg 2/1
  RF Loopback Select/1 -> RFA Rx Buffers/2(I/Q)
  RF Loopback Select1/1 -> RFB Rx Buffers/2(I/Q)
  RFB Inputs/2(I/Q) -> RFB Input Reg2/1
  RFC Inputs/2(I/Q) -> RFC Input Reg2/1
  RFD Inputs/2(I/Q) -> RFD Input Reg2/1
  RFB Input Reg2/1 -> RF Loopback Select1/2
  RFA Input Reg 2/1 -> RF Loopback Select/2
  TX RX Loopback Reg/1 -> RF Loopback Select/1, RF Loopback Select1/1, RF Loopback Select3/1, RF Loopback Select2/1
  RFA Input Reg 1/1 -> RFA Rx Buffers/1(RSSI)
  RFA Input Reg 3/1 -> RFA Rx Buffers/3(Addr)
  RFA Input Reg 4/1 -> RFA Rx Buffers/4(WE)
  RFA Input Reg 5/1 -> RFA Rx Buffers/5(EN)
  RFB Input Reg1/1 -> RFB Rx Buffers/1(RSSI)
  RFB Input Reg3/1 -> RFB Rx Buffers/3(Addr)
  RFB Input Reg4/1 -> RFB Rx Buffers/4(WE)
  RFB Input Reg5/1 -> RFB Rx Buffers/5(EN)
  tx output mux reg/1 -> RF Select/9
  tx output mux reg1/1 -> RF Select/8
  tx output mux reg2/1 -> RF Select/7
  tx output mux reg3/1 -> RF Select/6
  tx output mux reg4/1 -> RF Select/5
  tx output mux reg5/1 -> RF Select/4
  tx output mux reg6/1 -> RF Select/3
  tx output mux reg7/1 -> RF Select/2
  tx output mux reg8/1 -> RF Select/1
  tx output mux reg9/1 -> TX Output Select/1
  tx output mux reg10/1 -> TX Output Select/2
  TX Output Select/1 -> tx output mux reg11/1
  tx output mux reg11/1 -> transmit_running/1
  Convert3/1 -> tx output mux reg2/1
  RFC Input Reg1/1 -> RFC Rx Buffers/1(RSSI)
  RFC Input Reg3/1 -> RFC Rx Buffers/3(Addr)
  RFC Input Reg4/1 -> RFC Rx Buffers/4(WE)
  RFC Input Reg5/1 -> RFC Rx Buffers/5(EN)
  RFD Input Reg1/1 -> RFD Rx Buffers/1(RSSI)
  RFD Input Reg3/1 -> RFD Rx Buffers/3(Addr)
  RFD Input Reg4/1 -> RFD Rx Buffers/4(WE)
  RFD Input Reg5/1 -> RFD Rx Buffers/5(EN)
  RF Loopback Select3/1 -> RFC Rx Buffers/2(I/Q)
  RF Loopback Select2/1 -> RFD Rx Buffers/2(I/Q)
  RFC Input Reg2/1 -> RF Loopback Select3/2
  RFD Input Reg2/1 -> RF Loopback Select2/2

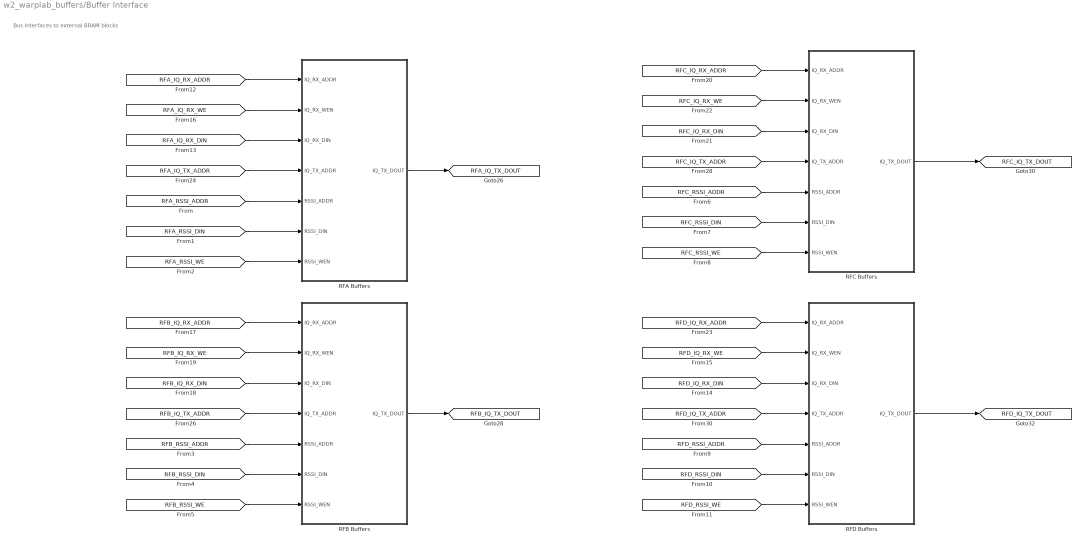
== system w2_warplab_buffers/Buffer Interface ==
  note: Bus Interfaces to external BRAM blocks
  RFA Buffers : Subsystem
  RFB Buffers : Subsystem
  RFC Buffers : Subsystem
  RFD Buffers : Subsystem
  tag scope: RFA_IQ_TX_DOUT=global, RFB_IQ_TX_DOUT=global, RFC_IQ_TX_DOUT=global, RFD_IQ_TX_DOUT=global
  wires:
  [RFA_RSSI_ADDR] -> RFA Buffers/5(RSSI_ADDR)
  [RFA_RSSI_DIN] -> RFA Buffers/6(RSSI_DIN)
  [RFA_RSSI_WE] -> RFA Buffers/7(RSSI_WEN)
  RFA Buffers/1(IQ_TX_DOUT) -> [RFA_IQ_TX_DOUT]
  [RFA_IQ_RX_ADDR] -> RFA Buffers/1(IQ_RX_ADDR)
  [RFA_IQ_RX_WE] -> RFA Buffers/2(IQ_RX_WEN)
  [RFA_IQ_RX_DIN] -> RFA Buffers/3(IQ_RX_DIN)
  [RFA_IQ_TX_ADDR] -> RFA Buffers/4(IQ_TX_ADDR)
  [RFB_IQ_RX_ADDR] -> RFB Buffers/1(IQ_RX_ADDR)
  [RFB_IQ_RX_WE] -> RFB Buffers/2(IQ_RX_WEN)
  [RFB_IQ_RX_DIN] -> RFB Buffers/3(IQ_RX_DIN)
  [RFB_IQ_TX_ADDR] -> RFB Buffers/4(IQ_TX_ADDR)
  [RFB_RSSI_ADDR] -> RFB Buffers/5(RSSI_ADDR)
  [RFB_RSSI_DIN] -> RFB Buffers/6(RSSI_DIN)
  [RFB_RSSI_WE] -> RFB Buffers/7(RSSI_WEN)
  RFB Buffers/1(IQ_TX_DOUT) -> [RFB_IQ_TX_DOUT]
  [RFC_IQ_RX_ADDR] -> RFC Buffers/1(IQ_RX_ADDR)
  [RFC_IQ_RX_WE] -> RFC Buffers/2(IQ_RX_WEN)
  [RFC_IQ_RX_DIN] -> RFC Buffers/3(IQ_RX_DIN)
  [RFC_IQ_TX_ADDR] -> RFC Buffers/4(IQ_TX_ADDR)
  [RFC_RSSI_ADDR] -> RFC Buffers/5(RSSI_ADDR)
  [RFC_RSSI_DIN] -> RFC Buffers/6(RSSI_DIN)
  [RFC_RSSI_WE] -> RFC Buffers/7(RSSI_WEN)
  RFC Buffers/1(IQ_TX_DOUT) -> [RFC_IQ_TX_DOUT]
  [RFD_IQ_RX_ADDR] -> RFD Buffers/1(IQ_RX_ADDR)
  [RFD_IQ_RX_WE] -> RFD Buffers/2(IQ_RX_WEN)
  [RFD_IQ_RX_DIN] -> RFD Buffers/3(IQ_RX_DIN)
  [RFD_IQ_TX_ADDR] -> RFD Buffers/4(IQ_TX_ADDR)
  [RFD_RSSI_ADDR] -> RFD Buffers/5(RSSI_ADDR)
  [RFD_RSSI_DIN] -> RFD Buffers/6(RSSI_DIN)
  [RFD_RSSI_WE] -> RFD Buffers/7(RSSI_WEN)
  RFD Buffers/1(IQ_TX_DOUT) -> [RFD_IQ_TX_DOUT]

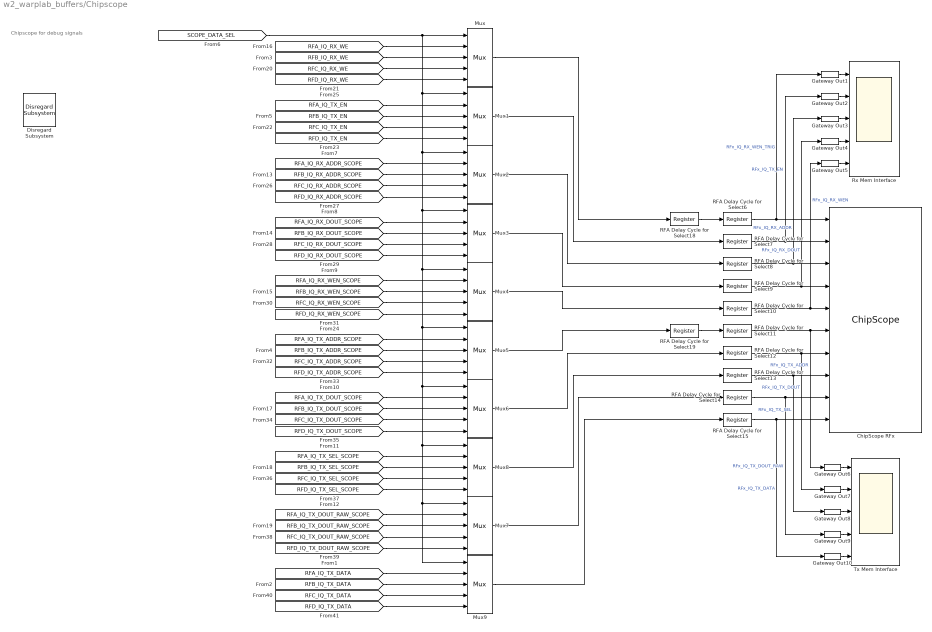
== system w2_warplab_buffers/Chipscope ==
  note: Chipscope for debug signals
  ChipScope RFx : xbsIndex_r4/ChipScope  num_trig_ports=2  current_port=0  show_trig_port=0  match_units=1  match_type=Basic  data_is_trigger=off  num_data_ports=8  data_depth=1024  SRL16s=on  add_bufg=on  match_type_t0=1  match_type_t1=1  match_type_t2=1  match_type_t3=1  match_type_t4=1  match_type_t5=1  match_type_t6=1  match_type_t7=1  match_type_t8=1  match_type_t9=1  match_type_t10=1  match_type_t11=1  match_type_t12=1  match_type_t13=1  match_type_t14=1  match_type_t15=1  match_units_t0=1  match_units_t1=1  match_units_t2=1  match_units_t3=1  match_units_t4=1  match_units_t5=1  match_units_t6=1  match_units_t7=1  match_units_t8=1  match_units_t9=1  match_units_t10=1  match_units_t11=1  match_units_t12=1  match_units_t13=1  match_units_t14=1  match_units_t15=1  dbl_ovrd=0  user_scan_chain=USER1  block_type=chipscope
      settings: infoedit="Enables run-time debugging and verification of signals by inserting ChipScope Pro ICON and ILA cores.<br><br>  Restrictions: <br>Only one ChipScope core can be instantiated in a System Generator design. A design or subsystem containing a ChipScope block must have at least one output port."
  Disregard Subsystem : xbsIndex_r4/Disregard Subsystem  Tag=discardX  block_type=disregard
  Gateway Out{1..10} (10 alike) : xbsIndex_r4/Gateway Out  inherit_from_input=off  hdl_port=off  timing_constraint=None  locs_specified=off  LOCs={}  UseAsDAC=off  DACChannel='1'  block_type=gatewayout
      settings: infoedit="Gateway out block.  Converts Xilinx fixed point inputs into ouputs of type Simulink integer, double, or fixed point.<P><P>Hardware notes:  In hardware these blocks become top level output ports or are discarded, depending on how they are configured."  block_version=10.1.2
  Mux{,1..9} (10 alike) : xbsIndex_r4/Mux  inputs=4  en=off  latency=0  precision=Full  arith_type=Unsigned  n_bits=16  bin_pt=14  quantization=Truncate  overflow=Wrap  dbl_ovrd=off  block_type=mux
  RFA Delay Cycle for Select{6..15,18..19} (12 alike) : xbsIndex_r4/Register  init=0  rst=off  en=off  dbl_ovrd=off  block_type=register
  Rx Mem Interface : Scope  NumInputPorts=5
      settings: TimeRange=70000  YMin=0~0~0~0~0  YMax=1~1~1~100~20000
  Tx Mem Interface : Scope  NumInputPorts=5
      settings: TimeRange=70000  YMin=0~0~0~0~0  YMax=1~1~1~100~20000  SaveName=ScopeData4
  wires:
  RFA Delay Cycle for Select18/1 -> RFA Delay Cycle for Select6/1
  RFA Delay Cycle for Select19/1 -> RFA Delay Cycle for Select11/1
  RFA Delay Cycle for Select6/1 -> ChipScope RFx/1, Gateway Out1/1  "RFx_IQ_RX_WEN_TRIG"
  RFA Delay Cycle for Select7/1 -> ChipScope RFx/2, Gateway Out2/1  "RFx_IQ_TX_EN"
  RFA Delay Cycle for Select8/1 -> ChipScope RFx/3, Gateway Out3/1  "RFx_IQ_RX_ADDR"
  RFA Delay Cycle for Select9/1 -> ChipScope RFx/4, Gateway Out4/1  "RFx_IQ_RX_DOUT"
  RFA Delay Cycle for Select10/1 -> ChipScope RFx/5, Gateway Out5/1  "RFx_IQ_RX_WEN"
  RFA Delay Cycle for Select11/1 -> ChipScope RFx/6, Gateway Out6/1  "RFx_IQ_TX_ADDR"
  RFA Delay Cycle for Select12/1 -> ChipScope RFx/7, Gateway Out7/1  "RFx_IQ_TX_DOUT"
  RFA Delay Cycle for Select13/1 -> ChipScope RFx/8, Gateway Out8/1  "RFx_IQ_TX_SEL"
  RFA Delay Cycle for Select14/1 -> ChipScope RFx/9, Gateway Out9/1  "RFx_IQ_TX_DOUT_RAW"
  RFA Delay Cycle for Select15/1 -> ChipScope RFx/10, Gateway Out10/1  "RFx_IQ_TX_DATA"
  [RFA_IQ_RX_WE] -> Mux/2
  [SCOPE_DATA_SEL] -> Mux/1, Mux1/1, Mux2/1, Mux3/1, Mux4/1, Mux5/1, Mux6/1, Mux8/1, Mux7/1, Mux9/1
  [RFB_IQ_RX_WE] -> Mux/3
  Mux/1 -> RFA Delay Cycle for Select18/1
  Mux1/1 -> RFA Delay Cycle for Select7/1
  Mux2/1 -> RFA Delay Cycle for Select8/1
  Mux3/1 -> RFA Delay Cycle for Select9/1
  Mux4/1 -> RFA Delay Cycle for Select10/1
  Mux5/1 -> RFA Delay Cycle for Select19/1
  Mux6/1 -> RFA Delay Cycle for Select12/1
  Mux8/1 -> RFA Delay Cycle for Select13/1
  Mux7/1 -> RFA Delay Cycle for Select14/1
  Mux9/1 -> RFA Delay Cycle for Select15/1
  [RFA_IQ_TX_EN] -> Mux1/2
  [RFB_IQ_TX_EN] -> Mux1/3
  [RFA_IQ_RX_ADDR_SCOPE] -> Mux2/2
  [RFB_IQ_RX_ADDR_SCOPE] -> Mux2/3
  [RFA_IQ_RX_DOUT_SCOPE] -> Mux3/2
  [RFB_IQ_RX_DOUT_SCOPE] -> Mux3/3
  [RFA_IQ_RX_WEN_SCOPE] -> Mux4/2
  [RFB_IQ_RX_WEN_SCOPE] -> Mux4/3
  [RFA_IQ_TX_ADDR_SCOPE] -> Mux5/2
  [RFB_IQ_TX_ADDR_SCOPE] -> Mux5/3
  [RFA_IQ_TX_DOUT_SCOPE] -> Mux6/2
  [RFB_IQ_TX_DOUT_SCOPE] -> Mux6/3
  [RFA_IQ_TX_SEL_SCOPE] -> Mux8/2
  [RFB_IQ_TX_SEL_SCOPE] -> Mux8/3
  [RFA_IQ_TX_DOUT_RAW_SCOPE] -> Mux7/2
  [RFB_IQ_TX_DOUT_RAW_SCOPE] -> Mux7/3
  [RFA_IQ_TX_DATA] -> Mux9/2
  [RFB_IQ_TX_DATA] -> Mux9/3
  [RFC_IQ_RX_WE] -> Mux/4
  [RFD_IQ_RX_WE] -> Mux/5
  [RFC_IQ_TX_EN] -> Mux1/4
  [RFD_IQ_TX_EN] -> Mux1/5
  [RFC_IQ_RX_ADDR_SCOPE] -> Mux2/4
  [RFD_IQ_RX_ADDR_SCOPE] -> Mux2/5
  [RFC_IQ_RX_DOUT_SCOPE] -> Mux3/4
  [RFD_IQ_RX_DOUT_SCOPE] -> Mux3/5
  [RFC_IQ_RX_WEN_SCOPE] -> Mux4/4
  [RFD_IQ_RX_WEN_SCOPE] -> Mux4/5
  [RFC_IQ_TX_ADDR_SCOPE] -> Mux5/4
  [RFD_IQ_TX_ADDR_SCOPE] -> Mux5/5
  [RFC_IQ_TX_DOUT_SCOPE] -> Mux6/4
  [RFD_IQ_TX_DOUT_SCOPE] -> Mux6/5
  [RFC_IQ_TX_SEL_SCOPE] -> Mux8/4
  [RFD_IQ_TX_SEL_SCOPE] -> Mux8/5
  [RFC_IQ_TX_DOUT_RAW_SCOPE] -> Mux7/4
  [RFD_IQ_TX_DOUT_RAW_SCOPE] -> Mux7/5
  [RFC_IQ_TX_DATA] -> Mux9/4
  [RFD_IQ_TX_DATA] -> Mux9/5
  Gateway Out1/1 -> Rx Mem Interface/1
  Gateway Out2/1 -> Rx Mem Interface/2
  Gateway Out3/1 -> Rx Mem Interface/3
  Gateway Out4/1 -> Rx Mem Interface/4
  Gateway Out5/1 -> Rx Mem Interface/5
  Gateway Out6/1 -> Tx Mem Interface/1
  Gateway Out7/1 -> Tx Mem Interface/2
  Gateway Out8/1 -> Tx Mem Interface/3
  Gateway Out9/1 -> Tx Mem Interface/4
  Gateway Out10/1 -> Tx Mem Interface/5
